simulink model "untitled3"  (R2022a)
settings: Solver=VariableStepAuto  StartTime=0.0  StopTime=10.0  RelTol=1e-3
undefined symbols (not defined in the file): rcosine
libraries: commrandsrc3 x1, commsink2 x1, commutil2 x1, dspsigops x1
settings Model: Creator=Administrator  LastModifiedBy=Administrator

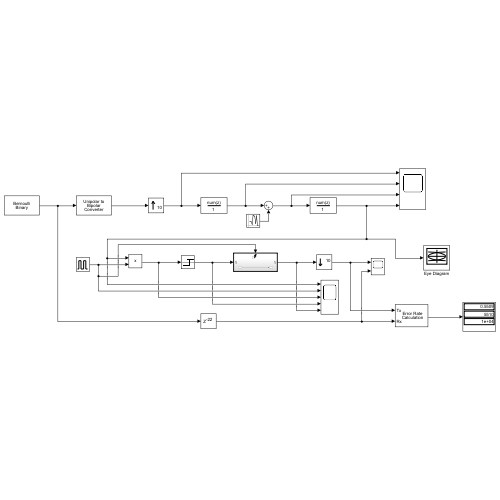
[thumbnail: Simulink's stored preview of the top-level diagram]
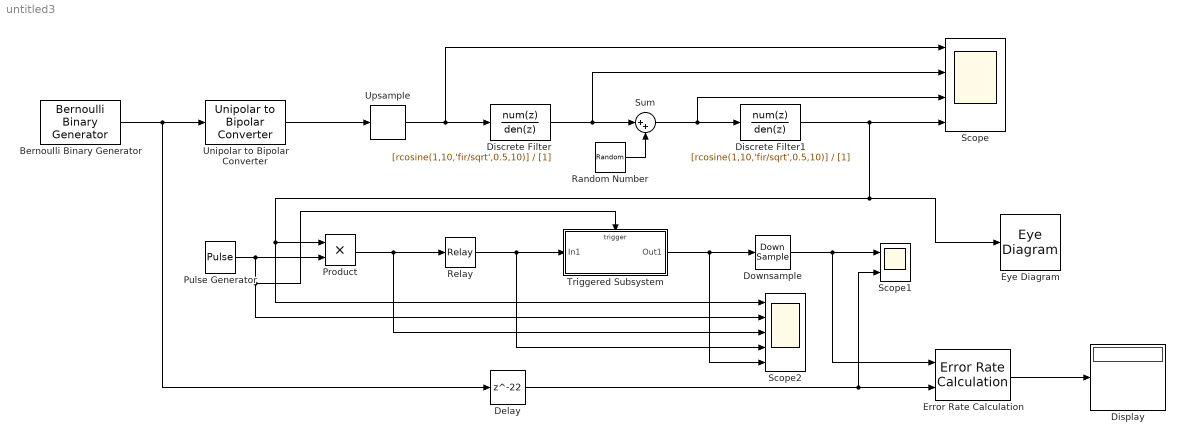
== system untitled3 ==
  Bernoulli Binary Generator : commrandsrc3/Bernoulli Binary Generator  ProbabilityOfZero=0.5  SeedSource=Auto  Seed=0  SampleTime=1/1000  SamplesPerFrame=1  OutputDataType=double  SimulateUsing=Interpreted execution
  Delay : Delay  DelayLength=22  InitialCondition=0
  Discrete Filter : DiscreteFilter  Numerator=[rcosine(1,10,'fir/sqrt',0.5,10)]  Denominator=[1]  SampleTime=1/10000
  Discrete Filter1 : DiscreteFilter  Numerator=[rcosine(1,10,'fir/sqrt',0.5,10)]  Denominator=[1]  SampleTime=1/10000
  Display : Display
  Downsample : DownSample  N=10
  Error Rate Calculation : commsink2/Error Rate Calculation  N=0  st_delay=0  cp_mode=Entire frame  subframe=[]  PMode=Port  WsName=ErrorVec  RsMode2=off  stop=off  numErr=100  maxBits=1e6
  Eye Diagram : EyeDiagram
  Product : Product
  Pulse Generator : DiscretePulseGenerator  PulseType=Time based  Period=0.001  PulseWidth=5
  Random Number : RandomNumber  SampleTime=0.1
  Relay : Relay
  Scope : Scope  NumInputPorts=4
  Scope1 : Scope  NumInputPorts=2
  Scope2 : Scope  NumInputPorts=5
  Sum : Sum  Inputs=|++
  Triggered Subsystem : Subsystem  TreatAsAtomicUnit=on
  Unipolar to Bipolar Converter : commutil2/Unipolar to Bipolar Converter  M=2  polarity=Positive  dataType=Inherit via internal rule
  Upsample : dspsigops/Upsample  N=10  phase=0  InputProcessing=Columns as channels (frame based)  RateOptions=Enforce single-rate processing  ic=0  mode=Unused parameter value
  wires:
  Bernoulli Binary Generator/1 -> Delay/1, Unipolar to Bipolar Converter/1
  Delay/1 -> Error Rate Calculation/2, Scope1/2
  Unipolar to Bipolar Converter/1 -> Upsample/1
  Random Number/1 -> Sum/2
  Upsample/1 -> Scope/1, Discrete Filter/1
  Discrete Filter/1 -> Scope/2, Sum/1
  Sum/1 -> Scope/3, Discrete Filter1/1
  Discrete Filter1/1 -> Eye Diagram/1, Product/1, Scope2/1, Scope/4
  Error Rate Calculation/1 -> Display/1
  Pulse Generator/1 -> Scope2/2, Triggered Subsystem/Trigger, Product/2
  Product/1 -> Scope2/3, Relay/1
  Relay/1 -> Scope2/4, Triggered Subsystem/1(In1)
  Triggered Subsystem/1(Out1) -> Scope2/5, Downsample/1
  Downsample/1 -> Error Rate Calculation/1, Scope1/1

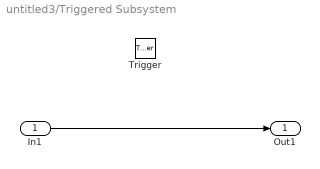
== system untitled3/Triggered Subsystem ==
  In1 : Inport
  Trigger : TriggerPort  VariantControl=(inherit)
  Out1 : Outport
  wires:
  In1/1 -> Out1/1
